simulink model "IEEE30_case"  (R2024b)
settings: Solver=FixedStepAuto  StartTime=0  StopTime=5  FixedStep=1e-7  RelTol=1e-3
values from neighbouring files (symbols this model uses):
  GFL_DFIG_7_C_bus = 0.08    [IEEE30_case_parameters.m]
  GFL_DFIG_7_D_mutual = 2.500000e+3    (= 2500)    [IEEE30_case_parameters.m]
  GFL_DFIG_7_f0 = 60    [IEEE30_case_parameters.m]
  GFL_DFIG_7_gPLLi = 3200    [IEEE30_case_parameters.m]
  GFL_DFIG_7_gPLLp = 650    [IEEE30_case_parameters.m]
  GFL_DFIG_7_H_WT = 0.4    [IEEE30_case_parameters.m]
  GFL_DFIG_7_Hg = 0.8    [IEEE30_case_parameters.m]
  GFL_DFIG_7_Igq_ref = 0    [IEEE30_case_parameters.m]
  GFL_DFIG_7_Ird_ref = 704.45696    [IEEE30_case_parameters.m]
  GFL_DFIG_7_KI_V = -300000    [IEEE30_case_parameters.m]
  GFL_DFIG_7_KP_V = -1000    [IEEE30_case_parameters.m]
  GFL_DFIG_7_Ksh = 1.254300e+4    (= 12543)    [IEEE30_case_parameters.m]
  GFL_DFIG_7_Lg = 0.000483    [IEEE30_case_parameters.m]
  GFL_DFIG_7_Lm_pu = 4    [IEEE30_case_parameters.m]
  GFL_DFIG_7_N = 100    [IEEE30_case_parameters.m]
  GFL_DFIG_7_p = 2    [IEEE30_case_parameters.m]
  GFL_DFIG_7_Pitch = 0    [IEEE30_case_parameters.m]
  GFL_DFIG_7_R = 44    [IEEE30_case_parameters.m]
  GFL_DFIG_7_Rg = 2.000000e-5    (= 2e-05)    [IEEE30_case_parameters.m]
  GFL_DFIG_7_rho = 1.225    [IEEE30_case_parameters.m]
  GFL_DFIG_7_rPLLi = 4500    [IEEE30_case_parameters.m]
  GFL_DFIG_7_rPLLp = 620    [IEEE30_case_parameters.m]
  GFL_DFIG_7_Rs_pu = 0.011    [IEEE30_case_parameters.m]
  GFL_DFIG_7_Sbase = 2.000000e+6    (= 2000000)    [IEEE30_case_parameters.m]
  GFL_DFIG_7_ugq_ref = 0    [IEEE30_case_parameters.m]
  GFL_DFIG_7_usd_ref = 0    [IEEE30_case_parameters.m]
  GFL_DFIG_7_Vbase = 690    [IEEE30_case_parameters.m]
  GFL_DFIG_7_Vdc_ref = 1200    [IEEE30_case_parameters.m]
  GFL_DFIG_7_wind = 12    [IEEE30_case_parameters.m]
  GFL_DFIG_7_wm_ref = 518.184209    [IEEE30_case_parameters.m]
  SG_D_13_D = 0.01056    [IEEE30_case_parameters.m]
  SG_D_13_EnableSaturation = 0    [IEEE30_case_parameters.m]
  SG_D_13_f0 = 60    [IEEE30_case_parameters.m]
  SG_D_13_H = 7.5    [IEEE30_case_parameters.m]
  SG_D_13_K_A = 20    [IEEE30_case_parameters.m]
  SG_D_13_K_E = 1.000000e+1    (= 10)    [IEEE30_case_parameters.m]
  SG_D_13_K_F = 2.363    [IEEE30_case_parameters.m]
  SG_D_13_K_s = 0.5    [IEEE30_case_parameters.m]
  SG_D_13_R_a = 0.001088    [IEEE30_case_parameters.m]
  SG_D_13_S_A = 1    [IEEE30_case_parameters.m]
  SG_D_13_S_B = 0.103    [IEEE30_case_parameters.m]
  SG_D_13_S_N = 10.659857    [IEEE30_case_parameters.m]
  SG_D_13_SpeedPara = 200    [IEEE30_case_parameters.m]
  SG_D_13_T_0 = 0.370163    [IEEE30_case_parameters.m]
  SG_D_13_T_1 = 0.3    [IEEE30_case_parameters.m]
  SG_D_13_T_2 = 0.05    [IEEE30_case_parameters.m]
  SG_D_13_T_3 = 0.02    [IEEE30_case_parameters.m]
  SG_D_13_T_4 = 0.005    [IEEE30_case_parameters.m]
  SG_D_13_T_A = 0.02    [IEEE30_case_parameters.m]
  SG_D_13_T_dd = 8.000000e+0    (= 8)    [IEEE30_case_parameters.m]
  SG_D_13_T_ddd = 0.04    [IEEE30_case_parameters.m]
  SG_D_13_T_E = 0.314    [IEEE30_case_parameters.m]
  SG_D_13_T_F = 0.35    [IEEE30_case_parameters.m]
  SG_D_13_T_qd = 0.8    [IEEE30_case_parameters.m]
  SG_D_13_T_qdd = 0.02    [IEEE30_case_parameters.m]
  SG_D_13_T_speed = 0.1    [IEEE30_case_parameters.m]
  SG_D_13_T_w = 0.5    [IEEE30_case_parameters.m]
  SG_D_13_V_ref = 1.696619    [IEEE30_case_parameters.m]
  SG_D_13_w_ref = 376.991118    [IEEE30_case_parameters.m]
  SG_D_13_x_d = 1.9    [IEEE30_case_parameters.m]
  SG_D_13_x_dd = 0.302    [IEEE30_case_parameters.m]
  SG_D_13_x_ddd = 0.204    [IEEE30_case_parameters.m]
  SG_D_13_x_l = 0.05    [IEEE30_case_parameters.m]
  SG_D_13_x_q = 1.3    [IEEE30_case_parameters.m]
  SG_D_13_x_qd = 0.5    [IEEE30_case_parameters.m]
  SG_D_13_x_qdd = 0.3    [IEEE30_case_parameters.m]
  SG_D_1_D = 0.01056    [IEEE30_case_parameters.m]
  SG_D_1_EnableSaturation = 0    [IEEE30_case_parameters.m]
  SG_D_1_f0 = 60    [IEEE30_case_parameters.m]
  SG_D_1_H = 7.5    [IEEE30_case_parameters.m]
  SG_D_1_K_A = 20    [IEEE30_case_parameters.m]
  SG_D_1_K_E = 1.000000e+1    (= 10)    [IEEE30_case_parameters.m]
  SG_D_1_K_F = 2.363    [IEEE30_case_parameters.m]
  SG_D_1_K_s = 0.5    [IEEE30_case_parameters.m]
  SG_D_1_R_a = 0.001088    [IEEE30_case_parameters.m]
  SG_D_1_S_A = 1    [IEEE30_case_parameters.m]
  SG_D_1_S_B = 0.103    [IEEE30_case_parameters.m]
  SG_D_1_S_N = 10.659857    [IEEE30_case_parameters.m]
  SG_D_1_SpeedPara = 200    [IEEE30_case_parameters.m]
  SG_D_1_T_0 = 0.259812    [IEEE30_case_parameters.m]
  SG_D_1_T_1 = 0.3    [IEEE30_case_parameters.m]
  SG_D_1_T_2 = 0.05    [IEEE30_case_parameters.m]
  SG_D_1_T_3 = 0.02    [IEEE30_case_parameters.m]
  SG_D_1_T_4 = 0.005    [IEEE30_case_parameters.m]
  SG_D_1_T_A = 0.02    [IEEE30_case_parameters.m]
  SG_D_1_T_dd = 8.000000e+0    (= 8)    [IEEE30_case_parameters.m]
  SG_D_1_T_ddd = 0.04    [IEEE30_case_parameters.m]
  SG_D_1_T_E = 0.314    [IEEE30_case_parameters.m]
  SG_D_1_T_F = 0.35    [IEEE30_case_parameters.m]
  SG_D_1_T_qd = 0.8    [IEEE30_case_parameters.m]
  SG_D_1_T_qdd = 0.02    [IEEE30_case_parameters.m]
  SG_D_1_T_speed = 0.1    [IEEE30_case_parameters.m]
  SG_D_1_T_w = 0.5    [IEEE30_case_parameters.m]
  SG_D_1_V_ref = 1.544107    [IEEE30_case_parameters.m]
  SG_D_1_w_ref = 376.991118    [IEEE30_case_parameters.m]
  SG_D_1_x_d = 1.9    [IEEE30_case_parameters.m]
  SG_D_1_x_dd = 0.302    [IEEE30_case_parameters.m]
  SG_D_1_x_ddd = 0.204    [IEEE30_case_parameters.m]
  SG_D_1_x_l = 0.05    [IEEE30_case_parameters.m]
  SG_D_1_x_q = 1.3    [IEEE30_case_parameters.m]
  SG_D_1_x_qd = 0.5    [IEEE30_case_parameters.m]
  SG_D_1_x_qdd = 0.3    [IEEE30_case_parameters.m]
  SG_D_22_D = 0.01056    [IEEE30_case_parameters.m]
  SG_D_22_EnableSaturation = 0    [IEEE30_case_parameters.m]
  SG_D_22_f0 = 60    [IEEE30_case_parameters.m]
  SG_D_22_H = 7.5    [IEEE30_case_parameters.m]
  SG_D_22_K_A = 20    [IEEE30_case_parameters.m]
  SG_D_22_K_E = 1.000000e+1    (= 10)    [IEEE30_case_parameters.m]
  SG_D_22_K_F = 2.363    [IEEE30_case_parameters.m]
  SG_D_22_K_s = 0.5    [IEEE30_case_parameters.m]
  SG_D_22_R_a = 0.001088    [IEEE30_case_parameters.m]
  SG_D_22_S_A = 1    [IEEE30_case_parameters.m]
  SG_D_22_S_B = 0.103    [IEEE30_case_parameters.m]
  SG_D_22_S_N = 10.659857    [IEEE30_case_parameters.m]
  SG_D_22_SpeedPara = 200    [IEEE30_case_parameters.m]
  SG_D_22_T_0 = 0.216121    [IEEE30_case_parameters.m]
  SG_D_22_T_1 = 0.3    [IEEE30_case_parameters.m]
  SG_D_22_T_2 = 0.05    [IEEE30_case_parameters.m]
  SG_D_22_T_3 = 0.02    [IEEE30_case_parameters.m]
  SG_D_22_T_4 = 0.005    [IEEE30_case_parameters.m]
  ... (+126 more)
(part 8 of 27)

== system IEEE30_case/AC_1/d_iq_line_2_5_block ==
  note: d_iq_line_2_5 in IEEE30_case
      | $1884.95559215388\,\mathrm{vq}_{\mathrm{bus},2}-94.2477796076938\,\mathrm{iq}_{\mathrm{line},2,5}-376.991118430775\,\mathrm{id}_{\mathrm{line},2,5}-1884.95559215388\,\mathrm{vq}_{\mathrm{bus},5}$
      | Automatically generated on 2025-11-01 18:41:07 .
  State_id_line_2_5_54524 : Inport
  State_iq_line_2_5_e8b89 : Inport  Port=2
  State_vq_bus_2_03b90 : Inport  Port=3
  State_vq_bus_5_87317 : Inport  Port=4
  Add_a371a : Sum
  Constant_-376.991118430775_afe3f : Constant  Value=-376.991118430775
  Constant_1884.95559215388_7223d : Constant  Value=1884.95559215388
  Constant_1884.95559215388_7e2ac : Constant  Value=1884.95559215388
  Constant_94.2477796076938_c5ea2 : Constant  Value=94.2477796076938
  Product_7cc1a : Product
  Product_8b282 : Product
  Product_c2d6a : Product
  Product_f29d2 : Product
  Subtract_19345 : Sum  Inputs=+-
  Subtract_26d55 : Sum  Inputs=+-
  Blockout_d_iq_line_2_5_eff7c : Outport
  wires:
  Constant_-376.991118430775_afe3f/1 -> Product_7cc1a/1
  Product_7cc1a/1 -> Subtract_26d55/1
  State_id_line_2_5_54524/1 -> Product_7cc1a/2
  Constant_94.2477796076938_c5ea2/1 -> Product_f29d2/1
  State_iq_line_2_5_e8b89/1 -> Product_f29d2/2
  Product_f29d2/1 -> Subtract_26d55/2
  State_vq_bus_2_03b90/1 -> Product_c2d6a/2
  Product_c2d6a/1 -> Add_a371a/2
  Constant_1884.95559215388_7223d/1 -> Product_c2d6a/1
  Subtract_26d55/1 -> Add_a371a/1
  Product_8b282/1 -> Subtract_19345/2
  Constant_1884.95559215388_7e2ac/1 -> Product_8b282/1
  State_vq_bus_5_87317/1 -> Product_8b282/2
  Add_a371a/1 -> Subtract_19345/1
  Subtract_19345/1 -> Blockout_d_iq_line_2_5_eff7c/1

== system IEEE30_case/AC_1/d_iq_line_2_6_block ==
  note: d_iq_line_2_6 in IEEE30_case
      | $2094.39510239319\,\mathrm{vq}_{\mathrm{bus},2}-125.663706143592\,\mathrm{iq}_{\mathrm{line},2,6}-376.991118430775\,\mathrm{id}_{\mathrm{line},2,6}-2094.39510239319\,\mathrm{vq}_{\mathrm{bus},6}$
      | Automatically generated on 2025-11-01 18:41:10 .
  State_id_line_2_6_7b42f : Inport
  State_iq_line_2_6_17b05 : Inport  Port=2
  State_vq_bus_2_0704f : Inport  Port=3
  State_vq_bus_6_e98dc : Inport  Port=4
  Add_94bf2 : Sum
  Constant_-376.991118430775_61c83 : Constant  Value=-376.991118430775
  Constant_125.663706143592_83d9a : Constant  Value=125.663706143592
  Constant_2094.39510239319_5703c : Constant  Value=2094.39510239319
  Constant_2094.39510239319_adbae : Constant  Value=2094.39510239319
  Product_1e63b : Product
  Product_508a7 : Product
  Product_89e1e : Product
  Product_db02a : Product
  Subtract_5e54d : Sum  Inputs=+-
  Subtract_f5901 : Sum  Inputs=+-
  Blockout_d_iq_line_2_6_890b3 : Outport
  wires:
  Constant_-376.991118430775_61c83/1 -> Product_508a7/1
  State_id_line_2_6_7b42f/1 -> Product_508a7/2
  Constant_125.663706143592_83d9a/1 -> Product_db02a/1
  Product_db02a/1 -> Subtract_f5901/2
  Product_89e1e/1 -> Add_94bf2/2
  Constant_2094.39510239319_5703c/1 -> Product_89e1e/1
  State_iq_line_2_6_17b05/1 -> Product_db02a/2
  Product_508a7/1 -> Subtract_f5901/1
  State_vq_bus_2_0704f/1 -> Product_89e1e/2
  Subtract_f5901/1 -> Add_94bf2/1
  Product_1e63b/1 -> Subtract_5e54d/2
  Constant_2094.39510239319_adbae/1 -> Product_1e63b/1
  Add_94bf2/1 -> Subtract_5e54d/1
  State_vq_bus_6_e98dc/1 -> Product_1e63b/2
  Subtract_5e54d/1 -> Blockout_d_iq_line_2_6_890b3/1

== system IEEE30_case/AC_1/d_iq_line_3_4_block ==
  note: d_iq_line_3_4 in IEEE30_case
      | $9424.77796076938\,\mathrm{vq}_{\mathrm{bus},3}-94.2477796076938\,\mathrm{iq}_{\mathrm{line},3,4}-376.991118430775\,\mathrm{id}_{\mathrm{line},3,4}-9424.77796076938\,\mathrm{vq}_{\mathrm{bus},4}$
      | Automatically generated on 2025-11-01 18:41:05 .
  State_id_line_3_4_c2377 : Inport
  State_iq_line_3_4_a2132 : Inport  Port=2
  State_vq_bus_3_53dc7 : Inport  Port=3
  State_vq_bus_4_f5988 : Inport  Port=4
  Add_93964 : Sum
  Constant_-376.991118430775_c7e30 : Constant  Value=-376.991118430775
  Constant_94.2477796076938_a3062 : Constant  Value=94.2477796076938
  Constant_9424.77796076938_25937 : Constant  Value=9424.77796076938
  Constant_9424.77796076938_71653 : Constant  Value=9424.77796076938
  Product_1bd2b : Product
  Product_9bcd3 : Product
  Product_bb908 : Product
  Product_e88d9 : Product
  Subtract_42a0d : Sum  Inputs=+-
  Subtract_80c72 : Sum  Inputs=+-
  Blockout_d_iq_line_3_4_9b5ec : Outport
  wires:
  Constant_-376.991118430775_c7e30/1 -> Product_9bcd3/1
  Constant_94.2477796076938_a3062/1 -> Product_1bd2b/1
  Product_1bd2b/1 -> Subtract_42a0d/2
  Product_9bcd3/1 -> Subtract_42a0d/1
  State_id_line_3_4_c2377/1 -> Product_9bcd3/2
  State_iq_line_3_4_a2132/1 -> Product_1bd2b/2
  Product_bb908/1 -> Add_93964/2
  Constant_9424.77796076938_71653/1 -> Product_bb908/1
  State_vq_bus_3_53dc7/1 -> Product_bb908/2
  Product_e88d9/1 -> Subtract_80c72/2
  Subtract_42a0d/1 -> Add_93964/1
  Constant_9424.77796076938_25937/1 -> Product_e88d9/1
  State_vq_bus_4_f5988/1 -> Product_e88d9/2
  Add_93964/1 -> Subtract_80c72/1
  Subtract_80c72/1 -> Blockout_d_iq_line_3_4_9b5ec/1

== system IEEE30_case/AC_1/d_iq_line_4_12_block ==
  note: d_iq_line_4_12 in IEEE30_case
      | $1449.96584011837\,\mathrm{vq}_{\mathrm{bus},4}-376.991118430775\,\mathrm{id}_{\mathrm{line},4,12}-1449.96584011837\,\mathrm{vq}_{\mathrm{bus},12}$
      | Automatically generated on 2025-11-01 18:41:30 .
  State_id_line_4_12_e9a32 : Inport
  State_vq_bus_12_318e0 : Inport  Port=2
  State_vq_bus_4_bbada : Inport  Port=3
  Add_42926 : Sum
  Constant_-376.991118430775_8ab2d : Constant  Value=-376.991118430775
  Constant_1449.96584011837_54b12 : Constant  Value=1449.96584011837
  Constant_1449.96584011837_d2e29 : Constant  Value=1449.96584011837
  Product_7ffdd : Product
  Product_e5260 : Product
  Product_e61c8 : Product
  Subtract_d7829 : Sum  Inputs=+-
  Blockout_d_iq_line_4_12_9b276 : Outport
  wires:
  Constant_-376.991118430775_8ab2d/1 -> Product_7ffdd/1
  Constant_1449.96584011837_54b12/1 -> Product_e5260/1
  Product_e5260/1 -> Subtract_d7829/2
  Product_7ffdd/1 -> Subtract_d7829/1
  State_id_line_4_12_e9a32/1 -> Product_7ffdd/2
  State_vq_bus_12_318e0/1 -> Product_e5260/2
  Product_e61c8/1 -> Add_42926/2
  Constant_1449.96584011837_d2e29/1 -> Product_e61c8/1
  Add_42926/1 -> Blockout_d_iq_line_4_12_9b276/1
  State_vq_bus_4_bbada/1 -> Product_e61c8/2
  Subtract_d7829/1 -> Add_42926/1

== system IEEE30_case/AC_1/d_iq_line_4_6_block ==
  note: d_iq_line_4_6 in IEEE30_case
      | $9424.77796076938\,\mathrm{vq}_{\mathrm{bus},4}-94.2477796076938\,\mathrm{iq}_{\mathrm{line},4,6}-376.991118430775\,\mathrm{id}_{\mathrm{line},4,6}-9424.77796076938\,\mathrm{vq}_{\mathrm{bus},6}$
      | Automatically generated on 2025-11-01 18:41:12 .
  State_id_line_4_6_aad9c : Inport
  State_iq_line_4_6_338ba : Inport  Port=2
  State_vq_bus_4_bd5e4 : Inport  Port=3
  State_vq_bus_6_b2fe0 : Inport  Port=4
  Add_f3899 : Sum
  Constant_-376.991118430775_1ade0 : Constant  Value=-376.991118430775
  Constant_94.2477796076938_b364f : Constant  Value=94.2477796076938
  Constant_9424.77796076938_20b18 : Constant  Value=9424.77796076938
  Constant_9424.77796076938_69e60 : Constant  Value=9424.77796076938
  Product_28995 : Product
  Product_5675d : Product
  Product_6de9b : Product
  Product_811d8 : Product
  Subtract_07f3b : Sum  Inputs=+-
  Subtract_17cad : Sum  Inputs=+-
  Blockout_d_iq_line_4_6_3cc9a : Outport
  wires:
  State_iq_line_4_6_338ba/1 -> Product_6de9b/2
  Constant_-376.991118430775_1ade0/1 -> Product_5675d/1
  Constant_94.2477796076938_b364f/1 -> Product_6de9b/1
  Product_6de9b/1 -> Subtract_07f3b/2
  State_id_line_4_6_aad9c/1 -> Product_5675d/2
  Product_5675d/1 -> Subtract_07f3b/1
  Constant_9424.77796076938_69e60/1 -> Product_28995/1
  State_vq_bus_4_bd5e4/1 -> Product_28995/2
  Subtract_07f3b/1 -> Add_f3899/1
  Product_28995/1 -> Add_f3899/2
  Product_811d8/1 -> Subtract_17cad/2
  Constant_9424.77796076938_20b18/1 -> Product_811d8/1
  State_vq_bus_6_b2fe0/1 -> Product_811d8/2
  Add_f3899/1 -> Subtract_17cad/1
  Subtract_17cad/1 -> Blockout_d_iq_line_4_6_3cc9a/1

== system IEEE30_case/AC_1/d_iq_line_5_7_block ==
  note: d_iq_line_5_7 in IEEE30_case
      | $3141.59265358979\,\mathrm{vq}_{\mathrm{bus},5}-157.07963267949\,\mathrm{iq}_{\mathrm{line},5,7}-376.991118430775\,\mathrm{id}_{\mathrm{line},5,7}-3141.59265358979\,\mathrm{vq}_{\mathrm{bus},7}$
      | Automatically generated on 2025-11-01 18:41:15 .
  State_id_line_5_7_c3a9a : Inport
  State_iq_line_5_7_98783 : Inport  Port=2
  State_vq_bus_5_129b8 : Inport  Port=3
  State_vq_bus_7_b0dc6 : Inport  Port=4
  Add_6172d : Sum
  Constant_-376.991118430775_516df : Constant  Value=-376.991118430775
  Constant_157.07963267949_263dc : Constant  Value=157.07963267949
  Constant_3141.59265358979_47382 : Constant  Value=3141.59265358979
  Constant_3141.59265358979_720d9 : Constant  Value=3141.59265358979
  Product_25a26 : Product
  Product_4ad97 : Product
  Product_59bd4 : Product
  Product_d4615 : Product
  Subtract_670ee : Sum  Inputs=+-
  Subtract_989a0 : Sum  Inputs=+-
  Blockout_d_iq_line_5_7_5e840 : Outport
  wires:
  Constant_-376.991118430775_516df/1 -> Product_4ad97/1
  Product_4ad97/1 -> Subtract_670ee/1
  State_id_line_5_7_c3a9a/1 -> Product_4ad97/2
  Constant_157.07963267949_263dc/1 -> Product_59bd4/1
  Product_59bd4/1 -> Subtract_670ee/2
  State_iq_line_5_7_98783/1 -> Product_59bd4/2
  Product_25a26/1 -> Add_6172d/2
  Constant_3141.59265358979_720d9/1 -> Product_25a26/1
  State_vq_bus_5_129b8/1 -> Product_25a26/2
  Subtract_670ee/1 -> Add_6172d/1
  Constant_3141.59265358979_47382/1 -> Product_d4615/1
  State_vq_bus_7_b0dc6/1 -> Product_d4615/2
  Add_6172d/1 -> Subtract_989a0/1
  Product_d4615/1 -> Subtract_989a0/2
  Subtract_989a0/1 -> Blockout_d_iq_line_5_7_5e840/1

== system IEEE30_case/AC_1/d_iq_line_6_10_block ==
  note: d_iq_line_6_10 in IEEE30_case
      | $673.198425769241\,\mathrm{vq}_{\mathrm{bus},6}-376.991118430775\,\mathrm{id}_{\mathrm{line},6,10}-673.198425769241\,\mathrm{vq}_{\mathrm{bus},10}$
      | Automatically generated on 2025-11-01 18:41:24 .
  State_id_line_6_10_fd3de : Inport
  State_vq_bus_10_9c824 : Inport  Port=2
  State_vq_bus_6_fa482 : Inport  Port=3
  Add_8fad6 : Sum
  Constant_-376.991118430775_b3dc4 : Constant  Value=-376.991118430775
  Constant_673.198425769241_7fad7 : Constant  Value=673.198425769241
  Constant_673.198425769241_d3814 : Constant  Value=673.198425769241
  Product_129d7 : Product
  Product_6bf2e : Product
  Product_9f14d : Product
  Subtract_2b990 : Sum  Inputs=+-
  Blockout_d_iq_line_6_10_02488 : Outport
  wires:
  Constant_-376.991118430775_b3dc4/1 -> Product_129d7/1
  Product_129d7/1 -> Subtract_2b990/1
  State_id_line_6_10_fd3de/1 -> Product_129d7/2
  Constant_673.198425769241_d3814/1 -> Product_9f14d/1
  Product_9f14d/1 -> Subtract_2b990/2
  State_vq_bus_10_9c824/1 -> Product_9f14d/2
  Product_6bf2e/1 -> Add_8fad6/2
  Constant_673.198425769241_7fad7/1 -> Product_6bf2e/1
  State_vq_bus_6_fa482/1 -> Product_6bf2e/2
  Subtract_2b990/1 -> Add_8fad6/1
  Add_8fad6/1 -> Blockout_d_iq_line_6_10_02488/1

== system IEEE30_case/AC_1/d_iq_line_6_28_block ==
  note: d_iq_line_6_28 in IEEE30_case
      | $6283.18530717959\,\mathrm{vq}_{\mathrm{bus},6}-125.663706143592\,\mathrm{iq}_{\mathrm{line},6,28}-376.991118430775\,\mathrm{id}_{\mathrm{line},6,28}-6283.18530717959\,\mathrm{vq}_{\mathrm{bus},28}$
      | Automatically generated on 2025-11-01 18:42:31 .
  State_id_line_6_28_8e443 : Inport
  State_iq_line_6_28_bd7e8 : Inport  Port=2
  State_vq_bus_28_c063c : Inport  Port=3
  State_vq_bus_6_177ff : Inport  Port=4
  Add_6d067 : Sum
  Constant_-376.991118430775_906bc : Constant  Value=-376.991118430775
  Constant_125.663706143592_e6af5 : Constant  Value=125.663706143592
  Constant_6283.18530717959_22793 : Constant  Value=6283.18530717959
  Constant_6283.18530717959_eb312 : Constant  Value=6283.18530717959
  Product_0abd7 : Product
  Product_128c9 : Product
  Product_5e22f : Product
  Product_646a6 : Product
  Subtract_5dc35 : Sum  Inputs=+-
  Subtract_e4d26 : Sum  Inputs=+-
  Blockout_d_iq_line_6_28_5907d : Outport
  wires:
  State_id_line_6_28_8e443/1 -> Product_128c9/2
  Constant_-376.991118430775_906bc/1 -> Product_128c9/1
  Constant_125.663706143592_e6af5/1 -> Product_646a6/1
  Product_646a6/1 -> Subtract_5dc35/2
  State_iq_line_6_28_bd7e8/1 -> Product_646a6/2
  Product_128c9/1 -> Subtract_5dc35/1
  Product_0abd7/1 -> Subtract_e4d26/2
  Constant_6283.18530717959_22793/1 -> Product_0abd7/1
  State_vq_bus_28_c063c/1 -> Product_0abd7/2
  Subtract_5dc35/1 -> Subtract_e4d26/1
  Product_5e22f/1 -> Add_6d067/2
  Constant_6283.18530717959_eb312/1 -> Product_5e22f/1
  State_vq_bus_6_177ff/1 -> Product_5e22f/2
  Subtract_e4d26/1 -> Add_6d067/1
  Add_6d067/1 -> Blockout_d_iq_line_6_28_5907d/1

== system IEEE30_case/AC_1/d_iq_line_6_7_block ==
  note: d_iq_line_6_7 in IEEE30_case
      | $4712.38898038469\,\mathrm{vq}_{\mathrm{bus},6}-141.371669411541\,\mathrm{iq}_{\mathrm{line},6,7}-376.991118430775\,\mathrm{id}_{\mathrm{line},6,7}-4712.38898038469\,\mathrm{vq}_{\mathrm{bus},7}$
      | Automatically generated on 2025-11-01 18:41:17 .
  State_id_line_6_7_667e6 : Inport
  State_iq_line_6_7_562f8 : Inport  Port=2
  State_vq_bus_6_83d07 : Inport  Port=3
  State_vq_bus_7_9b0dd : Inport  Port=4
  Add_794fe : Sum
  Constant_-376.991118430775_81a88 : Constant  Value=-376.991118430775
  Constant_141.371669411541_92a0d : Constant  Value=141.371669411541
  Constant_4712.38898038469_6f32c : Constant  Value=4712.38898038469
  Constant_4712.38898038469_e9fde : Constant  Value=4712.38898038469
  Product_190ff : Product
  Product_32f70 : Product
  Product_ab4c4 : Product
  Product_ee51e : Product
  Subtract_10fa6 : Sum  Inputs=+-
  Subtract_c84df : Sum  Inputs=+-
  Blockout_d_iq_line_6_7_6dbe9 : Outport
  wires:
  Constant_-376.991118430775_81a88/1 -> Product_32f70/1
  Product_32f70/1 -> Subtract_10fa6/1
  State_id_line_6_7_667e6/1 -> Product_32f70/2
  Constant_141.371669411541_92a0d/1 -> Product_ee51e/1
  Product_190ff/1 -> Add_794fe/2
  Constant_4712.38898038469_6f32c/1 -> Product_190ff/1
  State_iq_line_6_7_562f8/1 -> Product_ee51e/2
  State_vq_bus_6_83d07/1 -> Product_190ff/2
  Product_ee51e/1 -> Subtract_10fa6/2
  Subtract_10fa6/1 -> Add_794fe/1
  Product_ab4c4/1 -> Subtract_c84df/2
  Constant_4712.38898038469_e9fde/1 -> Product_ab4c4/1
  State_vq_bus_7_9b0dd/1 -> Product_ab4c4/2
  Add_794fe/1 -> Subtract_c84df/1
  Subtract_c84df/1 -> Blockout_d_iq_line_6_7_6dbe9/1

== system IEEE30_case/AC_1/d_iq_line_6_8_block ==
  note: d_iq_line_6_8 in IEEE30_case
      | $9424.77796076938\,\mathrm{vq}_{\mathrm{bus},6}-94.2477796076938\,\mathrm{iq}_{\mathrm{line},6,8}-376.991118430775\,\mathrm{id}_{\mathrm{line},6,8}-9424.77796076938\,\mathrm{vq}_{\mathrm{bus},8}$
      | Automatically generated on 2025-11-01 18:41:19 .
  State_id_line_6_8_d622b : Inport
  State_iq_line_6_8_6bc9f : Inport  Port=2
  State_vq_bus_6_241ca : Inport  Port=3
  State_vq_bus_8_0df72 : Inport  Port=4
  Add_b3718 : Sum
  Constant_-376.991118430775_fad48 : Constant  Value=-376.991118430775
  Constant_94.2477796076938_eb35d : Constant  Value=94.2477796076938
  Constant_9424.77796076938_61207 : Constant  Value=9424.77796076938
  Constant_9424.77796076938_d91cc : Constant  Value=9424.77796076938
  Product_9a554 : Product
  Product_cf133 : Product
  Product_e540a : Product
  Product_ed09e : Product
  Subtract_a6489 : Sum  Inputs=+-
  Subtract_b0ec5 : Sum  Inputs=+-
  Blockout_d_iq_line_6_8_b8ba9 : Outport
  wires:
  Constant_-376.991118430775_fad48/1 -> Product_cf133/1
  Constant_94.2477796076938_eb35d/1 -> Product_e540a/1
  Product_e540a/1 -> Subtract_b0ec5/2
  State_id_line_6_8_d622b/1 -> Product_cf133/2
  State_iq_line_6_8_6bc9f/1 -> Product_e540a/2
  Product_9a554/1 -> Add_b3718/2
  Constant_9424.77796076938_61207/1 -> Product_9a554/1
  Product_cf133/1 -> Subtract_b0ec5/1
  State_vq_bus_6_241ca/1 -> Product_9a554/2
  Subtract_b0ec5/1 -> Add_b3718/1
  Product_ed09e/1 -> Subtract_a6489/2
  Constant_9424.77796076938_d91cc/1 -> Product_ed09e/1
  State_vq_bus_8_0df72/1 -> Product_ed09e/2
  Add_b3718/1 -> Subtract_a6489/1
  Subtract_a6489/1 -> Blockout_d_iq_line_6_8_b8ba9/1

== system IEEE30_case/AC_1/d_iq_line_6_9_block ==
  note: d_iq_line_6_9 in IEEE30_case
      | $1795.19580205131\,\mathrm{vq}_{\mathrm{bus},6}-376.991118430775\,\mathrm{id}_{\mathrm{line},6,9}-1795.19580205131\,\mathrm{vq}_{\mathrm{bus},9}$
      | Automatically generated on 2025-11-01 18:41:22 .
  State_id_line_6_9_7cf57 : Inport
  State_vq_bus_6_65d52 : Inport  Port=2
  State_vq_bus_9_a086b : Inport  Port=3
  Add_f6946 : Sum
  Constant_-376.991118430775_59e94 : Constant  Value=-376.991118430775
  Constant_1795.19580205131_6c4f5 : Constant  Value=1795.19580205131
  Constant_1795.19580205131_bd9ec : Constant  Value=1795.19580205131
  Product_09b80 : Product
  Product_17dc1 : Product
  Product_908ab : Product
  Subtract_cd50a : Sum  Inputs=+-
  Blockout_d_iq_line_6_9_e28b1 : Outport
  wires:
  Constant_-376.991118430775_59e94/1 -> Product_17dc1/1
  Constant_1795.19580205131_6c4f5/1 -> Product_908ab/1
  Product_908ab/1 -> Add_f6946/2
  Product_17dc1/1 -> Add_f6946/1
  State_id_line_6_9_7cf57/1 -> Product_17dc1/2
  State_vq_bus_6_65d52/1 -> Product_908ab/2
  Product_09b80/1 -> Subtract_cd50a/2
  Constant_1795.19580205131_bd9ec/1 -> Product_09b80/1
  Subtract_cd50a/1 -> Blockout_d_iq_line_6_9_e28b1/1
  State_vq_bus_9_a086b/1 -> Product_09b80/2
  Add_f6946/1 -> Subtract_cd50a/1

== system IEEE30_case/AC_1/d_iq_line_8_28_block ==
  note: d_iq_line_8_28 in IEEE30_case
      | $1884.95559215388\,\mathrm{vq}_{\mathrm{bus},8}-113.097335529233\,\mathrm{iq}_{\mathrm{line},8,28}-376.991118430775\,\mathrm{id}_{\mathrm{line},8,28}-1884.95559215388\,\mathrm{vq}_{\mathrm{bus},28}$
      | Automatically generated on 2025-11-01 18:42:28 .
  State_id_line_8_28_812ec : Inport
  State_iq_line_8_28_65df2 : Inport  Port=2
  State_vq_bus_28_2fdab : Inport  Port=3
  State_vq_bus_8_f157d : Inport  Port=4
  Add_148f8 : Sum
  Constant_-376.991118430775_e146a : Constant  Value=-376.991118430775
  Constant_113.097335529233_20841 : Constant  Value=113.097335529233
  Constant_1884.95559215388_0a6d6 : Constant  Value=1884.95559215388
  Constant_1884.95559215388_3768c : Constant  Value=1884.95559215388
  Product_312c0 : Product
  Product_51235 : Product
  Product_960d5 : Product
  Product_b56d3 : Product
  Subtract_9c826 : Sum  Inputs=+-
  Subtract_beca7 : Sum  Inputs=+-
  Blockout_d_iq_line_8_28_1c551 : Outport
  wires:
  Constant_-376.991118430775_e146a/1 -> Product_51235/1
  Product_960d5/1 -> Subtract_9c826/2
  Constant_1884.95559215388_0a6d6/1 -> Product_960d5/1
  Product_51235/1 -> Subtract_beca7/1
  State_id_line_8_28_812ec/1 -> Product_51235/2
  Constant_113.097335529233_20841/1 -> Product_312c0/1
  Product_312c0/1 -> Subtract_beca7/2
  State_iq_line_8_28_65df2/1 -> Product_312c0/2
  State_vq_bus_28_2fdab/1 -> Product_960d5/2
  Subtract_beca7/1 -> Subtract_9c826/1
  Product_b56d3/1 -> Add_148f8/2
  Constant_1884.95559215388_3768c/1 -> Product_b56d3/1
  State_vq_bus_8_f157d/1 -> Product_b56d3/2
  Subtract_9c826/1 -> Add_148f8/1
  Add_148f8/1 -> Blockout_d_iq_line_8_28_1c551/1

== system IEEE30_case/AC_1/d_iq_line_9_10_block ==
  note: d_iq_line_9_10 in IEEE30_case
      | $3427.19198573432\,\mathrm{vq}_{\mathrm{bus},9}-376.991118430775\,\mathrm{id}_{\mathrm{line},9,10}-3427.19198573432\,\mathrm{vq}_{\mathrm{bus},10}$
      | Automatically generated on 2025-11-01 18:41:28 .
  State_id_line_9_10_9405b : Inport
  State_vq_bus_10_72139 : Inport  Port=2
  State_vq_bus_9_3ff0d : Inport  Port=3
  Add_264a1 : Sum
  Constant_-376.991118430775_5d75f : Constant  Value=-376.991118430775
  Constant_3427.19198573432_1f815 : Constant  Value=3427.19198573432
  Constant_3427.19198573432_58760 : Constant  Value=3427.19198573432
  Product_adb61 : Product
  Product_c8172 : Product
  Product_ef6f6 : Product
  Subtract_5c677 : Sum  Inputs=+-
  Blockout_d_iq_line_9_10_d1a46 : Outport
  wires:
  State_vq_bus_9_3ff0d/1 -> Product_c8172/2
  Constant_-376.991118430775_5d75f/1 -> Product_ef6f6/1
  Product_c8172/1 -> Add_264a1/2
  Product_ef6f6/1 -> Subtract_5c677/1
  Constant_3427.19198573432_1f815/1 -> Product_c8172/1
  State_id_line_9_10_9405b/1 -> Product_ef6f6/2
  Constant_3427.19198573432_58760/1 -> Product_adb61/1
  State_vq_bus_10_72139/1 -> Product_adb61/2
  Product_adb61/1 -> Subtract_5c677/2
  Subtract_5c677/1 -> Add_264a1/1
  Add_264a1/1 -> Blockout_d_iq_line_9_10_d1a46/1

== system IEEE30_case/AC_1/d_iq_line_9_11_block ==
  note: d_iq_line_9_11 in IEEE30_case
      | $1795.19580205131\,\mathrm{vq}_{\mathrm{bus},9}-376.991118430775\,\mathrm{id}_{\mathrm{line},9,11}-1795.19580205131\,\mathrm{vq}_{\mathrm{bus},11}$
      | Automatically generated on 2025-11-01 18:41:26 .
  State_id_line_9_11_716ef : Inport
  State_vq_bus_11_310c2 : Inport  Port=2
  State_vq_bus_9_0d25d : Inport  Port=3
  Add_3daa9 : Sum
  Constant_-376.991118430775_ec185 : Constant  Value=-376.991118430775
  Constant_1795.19580205131_3f8cc : Constant  Value=1795.19580205131
  Constant_1795.19580205131_4c27b : Constant  Value=1795.19580205131
  Product_0918f : Product
  Product_28f02 : Product
  Product_341b4 : Product
  Subtract_55c47 : Sum  Inputs=+-
  Blockout_d_iq_line_9_11_ec45f : Outport
  wires:
  Constant_-376.991118430775_ec185/1 -> Product_0918f/1
  Product_0918f/1 -> Subtract_55c47/1
  State_id_line_9_11_716ef/1 -> Product_0918f/2
  Constant_1795.19580205131_3f8cc/1 -> Product_28f02/1
  Product_28f02/1 -> Subtract_55c47/2
  Product_341b4/1 -> Add_3daa9/2
  Constant_1795.19580205131_4c27b/1 -> Product_341b4/1
  State_vq_bus_11_310c2/1 -> Product_28f02/2
  State_vq_bus_9_0d25d/1 -> Product_341b4/2
  Subtract_55c47/1 -> Add_3daa9/1
  Add_3daa9/1 -> Blockout_d_iq_line_9_11_ec45f/1

== system IEEE30_case/AC_1/d_iq_load_10_block ==
  note: d_iq_load_10 in IEEE30_case
      | $73.2156181903037\,\mathrm{vq}_{\mathrm{bus},10}-1093.27424344925\,\mathrm{iq}_{\mathrm{load},10}-376.991118430775\,\mathrm{id}_{\mathrm{load},10}$
      | Automatically generated on 2025-11-01 18:40:26 .
  State_id_load_10_13915 : Inport
  State_iq_load_10_267fb : Inport  Port=2
  State_vq_bus_10_c6f4b : Inport  Port=3
  Add_9bcc7 : Sum
  Constant_-376.991118430775_f4f50 : Constant  Value=-376.991118430775
  Constant_1093.27424344925_5db7f : Constant  Value=1093.27424344925
  Constant_73.2156181903037_815ec : Constant  Value=73.2156181903037
  Product_7e589 : Product
  Product_b1673 : Product
  Product_faef5 : Product
  Subtract_39713 : Sum  Inputs=+-
  Blockout_d_iq_load_10_a5f74 : Outport
  wires:
  Constant_-376.991118430775_f4f50/1 -> Product_faef5/1
  Constant_73.2156181903037_815ec/1 -> Product_b1673/1
  State_id_load_10_13915/1 -> Product_faef5/2
  Constant_1093.27424344925_5db7f/1 -> Product_7e589/1
  Product_7e589/1 -> Subtract_39713/2
  State_iq_load_10_267fb/1 -> Product_7e589/2
  Product_faef5/1 -> Subtract_39713/1
  State_vq_bus_10_c6f4b/1 -> Product_b1673/2
  Subtract_39713/1 -> Add_9bcc7/1
  Product_b1673/1 -> Add_9bcc7/2
  Add_9bcc7/1 -> Blockout_d_iq_load_10_a5f74/1

== system IEEE30_case/AC_1/d_iq_load_12_block ==
  note: d_iq_load_12 in IEEE30_case
      | $94.0406333232708\,\mathrm{vq}_{\mathrm{bus},12}-562.973403523291\,\mathrm{iq}_{\mathrm{load},12}-376.991118430775\,\mathrm{id}_{\mathrm{load},12}$
      | Automatically generated on 2025-11-01 18:40:28 .
  State_id_load_12_a9fac : Inport
  State_iq_load_12_0eed2 : Inport  Port=2
  State_vq_bus_12_ac2a3 : Inport  Port=3
  Add_91925 : Sum
  Constant_-376.991118430775_6100e : Constant  Value=-376.991118430775
  Constant_562.973403523291_a5745 : Constant  Value=562.973403523291
  Constant_94.0406333232708_6cdec : Constant  Value=94.0406333232708
  Product_cf934 : Product
  Product_d0b54 : Product
  Product_e8b5c : Product
  Subtract_c298b : Sum  Inputs=+-
  Blockout_d_iq_load_12_fd87b : Outport
  wires:
  Constant_-376.991118430775_6100e/1 -> Product_e8b5c/1
  Constant_562.973403523291_a5745/1 -> Product_d0b54/1
  Product_d0b54/1 -> Subtract_c298b/2
  State_id_load_12_a9fac/1 -> Product_e8b5c/2
  State_iq_load_12_0eed2/1 -> Product_d0b54/2
  Product_e8b5c/1 -> Subtract_c298b/1
  Constant_94.0406333232708_6cdec/1 -> Product_cf934/1
  State_vq_bus_12_ac2a3/1 -> Product_cf934/2
  Subtract_c298b/1 -> Add_91925/1
  Product_cf934/1 -> Add_91925/2
  Add_91925/1 -> Blockout_d_iq_load_12_fd87b/1

== system IEEE30_case/AC_1/d_iq_load_14_block ==
  note: d_iq_load_14 in IEEE30_case
      | $101.272894526084\,\mathrm{vq}_{\mathrm{bus},14}-1460.84058391925\,\mathrm{iq}_{\mathrm{load},14}-376.991118430775\,\mathrm{id}_{\mathrm{load},14}$
      | Automatically generated on 2025-11-01 18:40:31 .
  State_id_load_14_258e7 : Inport
  State_iq_load_14_32f4c : Inport  Port=2
  State_vq_bus_14_0c5a3 : Inport  Port=3
  Add_63ca6 : Sum
  Constant_-376.991118430775_c30c3 : Constant  Value=-376.991118430775
  Constant_101.272894526084_db1b1 : Constant  Value=101.272894526084
  Constant_1460.84058391925_06af2 : Constant  Value=1460.84058391925
  Product_91f16 : Product
  Product_969e2 : Product
  Product_a0568 : Product
  Subtract_fed73 : Sum  Inputs=+-
  Blockout_d_iq_load_14_e1c59 : Outport
  wires:
  State_id_load_14_258e7/1 -> Product_969e2/2
  Constant_-376.991118430775_c30c3/1 -> Product_969e2/1
  Constant_1460.84058391925_06af2/1 -> Product_91f16/1
  Product_91f16/1 -> Subtract_fed73/2
  State_iq_load_14_32f4c/1 -> Product_91f16/2
  Product_969e2/1 -> Subtract_fed73/1
  Constant_101.272894526084_db1b1/1 -> Product_a0568/1
  State_vq_bus_14_0c5a3/1 -> Product_a0568/2
  Subtract_fed73/1 -> Add_63ca6/1
  Product_a0568/1 -> Add_63ca6/2
  Add_63ca6/1 -> Blockout_d_iq_load_14_e1c59/1

== system IEEE30_case/AC_1/d_iq_load_15_block ==
  note: d_iq_load_15 in IEEE30_case
      | $115.335827789783\,\mathrm{vq}_{\mathrm{bus},15}-1236.53086845294\,\mathrm{iq}_{\mathrm{load},15}-376.991118430775\,\mathrm{id}_{\mathrm{load},15}$
      | Automatically generated on 2025-11-01 18:40:33 .
  State_id_load_15_529a5 : Inport
  State_iq_load_15_0f08a : Inport  Port=2
  State_vq_bus_15_9de62 : Inport  Port=3
  Add_cd18a : Sum
  Constant_-376.991118430775_b8f9e : Constant  Value=-376.991118430775
  Constant_115.335827789783_f0de2 : Constant  Value=115.335827789783
  Constant_1236.53086845294_ddcf3 : Constant  Value=1236.53086845294
  Product_24c1c : Product
  Product_e4fc8 : Product
  Product_f8424 : Product
  Subtract_891f8 : Sum  Inputs=+-
  Blockout_d_iq_load_15_d1c82 : Outport
  wires:
  Constant_-376.991118430775_b8f9e/1 -> Product_f8424/1
  State_id_load_15_529a5/1 -> Product_f8424/2
  Constant_1236.53086845294_ddcf3/1 -> Product_24c1c/1
  Product_24c1c/1 -> Subtract_891f8/2
  State_iq_load_15_0f08a/1 -> Product_24c1c/2
  Product_f8424/1 -> Subtract_891f8/1
  Constant_115.335827789783_f0de2/1 -> Product_e4fc8/1
  State_vq_bus_15_9de62/1 -> Product_e4fc8/2
  Subtract_891f8/1 -> Add_cd18a/1
  Product_e4fc8/1 -> Add_cd18a/2
  Add_cd18a/1 -> Blockout_d_iq_load_15_d1c82/1

== system IEEE30_case/AC_1/d_iq_load_16_block ==
  note: d_iq_load_16 in IEEE30_case
      | $33.9601202098734\,\mathrm{vq}_{\mathrm{bus},16}-733.038285837618\,\mathrm{iq}_{\mathrm{load},16}-376.991118430775\,\mathrm{id}_{\mathrm{load},16}$
      | Automatically generated on 2025-11-01 18:40:35 .
  State_id_load_16_bee16 : Inport
  State_iq_load_16_5f7c5 : Inport  Port=2
  State_vq_bus_16_c51f8 : Inport  Port=3
  Add_8dc90 : Sum
  Constant_-376.991118430775_4be04 : Constant  Value=-376.991118430775
  Constant_33.9601202098734_a71af : Constant  Value=33.9601202098734
  Constant_733.038285837618_846d7 : Constant  Value=733.038285837618
  Product_11f64 : Product
  Product_a999c : Product
  Product_ec6fc : Product
  Subtract_5712a : Sum  Inputs=+-
  Blockout_d_iq_load_16_0762f : Outport
  wires:
  Constant_-376.991118430775_4be04/1 -> Product_a999c/1
  Constant_33.9601202098734_a71af/1 -> Product_ec6fc/1
  State_id_load_16_bee16/1 -> Product_a999c/2
  Constant_733.038285837618_846d7/1 -> Product_11f64/1
  Product_11f64/1 -> Subtract_5712a/2
  State_iq_load_16_5f7c5/1 -> Product_11f64/2
  Product_a999c/1 -> Subtract_5712a/1
  State_vq_bus_16_c51f8/1 -> Product_ec6fc/2
  Subtract_5712a/1 -> Add_8dc90/1
  Product_ec6fc/1 -> Add_8dc90/2
  Add_8dc90/1 -> Blockout_d_iq_load_16_0762f/1

== system IEEE30_case/AC_1/d_iq_load_17_block ==
  note: d_iq_load_17 in IEEE30_case
      | $78.0853999068988\,\mathrm{vq}_{\mathrm{bus},17}-584.986218254651\,\mathrm{iq}_{\mathrm{load},17}-376.991118430775\,\mathrm{id}_{\mathrm{load},17}$
      | Automatically generated on 2025-11-01 18:40:37 .
  State_id_load_17_33982 : Inport
  State_iq_load_17_00d7f : Inport  Port=2
  State_vq_bus_17_aeaf0 : Inport  Port=3
  Add_f7430 : Sum
  Constant_-376.991118430775_351de : Constant  Value=-376.991118430775
  Constant_584.986218254651_41463 : Constant  Value=584.986218254651
  Constant_78.0853999068988_2afd1 : Constant  Value=78.0853999068988
  Product_19578 : Product
  Product_29a69 : Product
  Product_dc837 : Product
  Subtract_de1c4 : Sum  Inputs=+-
  Blockout_d_iq_load_17_3c8b9 : Outport
  wires:
  Constant_-376.991118430775_351de/1 -> Product_29a69/1
  Constant_584.986218254651_41463/1 -> Product_dc837/1
  Product_dc837/1 -> Subtract_de1c4/2
  State_id_load_17_33982/1 -> Product_29a69/2
  State_iq_load_17_00d7f/1 -> Product_dc837/2
  Product_29a69/1 -> Subtract_de1c4/1
  Constant_78.0853999068988_2afd1/1 -> Product_19578/1
  State_vq_bus_17_aeaf0/1 -> Product_19578/2
  Subtract_de1c4/1 -> Add_f7430/1
  Product_19578/1 -> Add_f7430/2
  Add_f7430/1 -> Blockout_d_iq_load_17_3c8b9/1

== system IEEE30_case/AC_1/d_iq_load_18_block ==
  note: d_iq_load_18 in IEEE30_case
      | $49.3520450041255\,\mathrm{vq}_{\mathrm{bus},18}-1340.41286553164\,\mathrm{iq}_{\mathrm{load},18}-376.991118430775\,\mathrm{id}_{\mathrm{load},18}$
      | Automatically generated on 2025-11-01 18:40:39 .
  State_id_load_18_cc435 : Inport
  State_iq_load_18_d8478 : Inport  Port=2
  State_vq_bus_18_1cdbe : Inport  Port=3
  Add_6fb2f : Sum
  Constant_-376.991118430775_f2fe2 : Constant  Value=-376.991118430775
  Constant_1340.41286553164_f73e8 : Constant  Value=1340.41286553164
  Constant_49.3520450041255_95a9c : Constant  Value=49.3520450041255
  Product_979f9 : Product
  Product_a76e6 : Product
  Product_ccd50 : Product
  Subtract_1e928 : Sum  Inputs=+-
  Blockout_d_iq_load_18_ea1d4 : Outport
  wires:
  State_id_load_18_cc435/1 -> Product_979f9/2
  Constant_-376.991118430775_f2fe2/1 -> Product_979f9/1
  Constant_1340.41286553164_f73e8/1 -> Product_ccd50/1
  Product_ccd50/1 -> Subtract_1e928/2
  State_iq_load_18_d8478/1 -> Product_ccd50/2
  Product_979f9/1 -> Subtract_1e928/1
  Constant_49.3520450041255_95a9c/1 -> Product_a76e6/1
  State_vq_bus_18_1cdbe/1 -> Product_a76e6/2
  Subtract_1e928/1 -> Add_6fb2f/1
  Product_a76e6/1 -> Add_6fb2f/2
  Add_6fb2f/1 -> Blockout_d_iq_load_18_ea1d4/1

== system IEEE30_case/AC_1/d_iq_load_19_block ==
  note: d_iq_load_19 in IEEE30_case
      | $121.151749063551\,\mathrm{vq}_{\mathrm{bus},19}-1053.35753679187\,\mathrm{iq}_{\mathrm{load},19}-376.991118430775\,\mathrm{id}_{\mathrm{load},19}$
      | Automatically generated on 2025-11-01 18:40:41 .
  State_id_load_19_a4f80 : Inport
  State_iq_load_19_a3943 : Inport  Port=2
  State_vq_bus_19_94ea2 : Inport  Port=3
  Add_410b9 : Sum
  Constant_-376.991118430775_f8b2f : Constant  Value=-376.991118430775
  Constant_1053.35753679187_737a4 : Constant  Value=1053.35753679187
  Constant_121.151749063551_5e61c : Constant  Value=121.151749063551
  Product_09819 : Product
  Product_8d40b : Product
  Product_8ed21 : Product
  Subtract_dd1ff : Sum  Inputs=+-
  Blockout_d_iq_load_19_8f082 : Outport
  wires:
  Constant_-376.991118430775_f8b2f/1 -> Product_8d40b/1
  State_id_load_19_a4f80/1 -> Product_8d40b/2
  Constant_1053.35753679187_737a4/1 -> Product_8ed21/1
  Product_8ed21/1 -> Subtract_dd1ff/2
  State_iq_load_19_a3943/1 -> Product_8ed21/2
  Product_8d40b/1 -> Subtract_dd1ff/1
  Constant_121.151749063551_5e61c/1 -> Product_09819/1
  State_vq_bus_19_94ea2/1 -> Product_09819/2
  Subtract_dd1ff/1 -> Add_410b9/1
  Product_09819/1 -> Add_410b9/2
  Add_410b9/1 -> Blockout_d_iq_load_19_8f082/1

== system IEEE30_case/AC_1/d_iq_load_20_block ==
  note: d_iq_load_20 in IEEE30_case
      | $30.5607236833912\,\mathrm{vq}_{\mathrm{bus},20}-1184.82922935387\,\mathrm{iq}_{\mathrm{load},20}-376.991118430775\,\mathrm{id}_{\mathrm{load},20}$
      | Automatically generated on 2025-11-01 18:40:43 .
  State_id_load_20_a93db : Inport
  State_iq_load_20_f0103 : Inport  Port=2
  State_vq_bus_20_5757f : Inport  Port=3
  Add_5fbfa : Sum
  Constant_-376.991118430775_98607 : Constant  Value=-376.991118430775
  Constant_1184.82922935387_99242 : Constant  Value=1184.82922935387
  Constant_30.5607236833912_655b2 : Constant  Value=30.5607236833912
  Product_1073e : Product
  Product_bcc77 : Product
  Product_fabfb : Product
  Subtract_cfad3 : Sum  Inputs=+-
  Blockout_d_iq_load_20_f0a03 : Outport
  wires:
  Constant_-376.991118430775_98607/1 -> Product_fabfb/1
  Constant_30.5607236833912_655b2/1 -> Product_bcc77/1
  State_id_load_20_a93db/1 -> Product_fabfb/2
  Constant_1184.82922935387_99242/1 -> Product_1073e/1
  Product_1073e/1 -> Subtract_cfad3/2
  Product_fabfb/1 -> Subtract_cfad3/1
  State_iq_load_20_f0103/1 -> Product_1073e/2
  State_vq_bus_20_5757f/1 -> Product_bcc77/2
  Subtract_cfad3/1 -> Add_5fbfa/1
  Product_bcc77/1 -> Add_5fbfa/2
  Add_5fbfa/1 -> Blockout_d_iq_load_20_f0a03/1

== system IEEE30_case/AC_1/d_iq_load_21_block ==
  note: d_iq_load_21 in IEEE30_case
      | $147.248668081812\,\mathrm{vq}_{\mathrm{bus},21}-589.048622548086\,\mathrm{iq}_{\mathrm{load},21}-376.991118430775\,\mathrm{id}_{\mathrm{load},21}$
      | Automatically generated on 2025-11-01 18:40:45 .
  State_id_load_21_1a39e : Inport
  State_iq_load_21_200f9 : Inport  Port=2
  State_vq_bus_21_cc767 : Inport  Port=3
  Add_47351 : Sum
  Constant_-376.991118430775_620ea : Constant  Value=-376.991118430775
  Constant_147.248668081812_ce267 : Constant  Value=147.248668081812
  Constant_589.048622548086_e8725 : Constant  Value=589.048622548086
  Product_409a9 : Product
  Product_8acc8 : Product
  Product_f535b : Product
  Subtract_8b118 : Sum  Inputs=+-
  Blockout_d_iq_load_21_5945b : Outport
  wires:
  Constant_-376.991118430775_620ea/1 -> Product_8acc8/1
  Constant_589.048622548086_e8725/1 -> Product_409a9/1
  Product_409a9/1 -> Subtract_8b118/2
  State_id_load_21_1a39e/1 -> Product_8acc8/2
  State_iq_load_21_200f9/1 -> Product_409a9/2
  Product_8acc8/1 -> Subtract_8b118/1
  Constant_147.248668081812_ce267/1 -> Product_f535b/1
  State_vq_bus_21_cc767/1 -> Product_f535b/2
  Subtract_8b118/1 -> Add_47351/1
  Product_f535b/1 -> Add_47351/2
  Add_47351/1 -> Blockout_d_iq_load_21_5945b/1

== system IEEE30_case/AC_1/d_iq_load_23_block ==
  note: d_iq_load_23 in IEEE30_case
      | $30.159289474462\,\mathrm{vq}_{\mathrm{bus},23}-753.98223686155\,\mathrm{iq}_{\mathrm{load},23}-376.991118430775\,\mathrm{id}_{\mathrm{load},23}$
      | Automatically generated on 2025-11-01 18:40:47 .
  State_id_load_23_359e1 : Inport
  State_iq_load_23_3c73d : Inport  Port=2
  State_vq_bus_23_fbc77 : Inport  Port=3
  Add_6b46f : Sum
  Constant_-376.991118430775_dc465 : Constant  Value=-376.991118430775
  Constant_30.159289474462_b946c : Constant  Value=30.159289474462
  Constant_753.98223686155_8a743 : Constant  Value=753.98223686155
  Product_11717 : Product
  Product_6b2be : Product
  Product_fb170 : Product
  Subtract_657dd : Sum  Inputs=+-
  Blockout_d_iq_load_23_36f94 : Outport
  wires:
  State_id_load_23_359e1/1 -> Product_11717/2
  Constant_-376.991118430775_dc465/1 -> Product_11717/1
  Constant_753.98223686155_8a743/1 -> Product_6b2be/1
  Product_6b2be/1 -> Subtract_657dd/2
  State_iq_load_23_3c73d/1 -> Product_6b2be/2
  Product_11717/1 -> Subtract_657dd/1
  Constant_30.159289474462_b946c/1 -> Product_fb170/1
  State_vq_bus_23_fbc77/1 -> Product_fb170/2
  Subtract_657dd/1 -> Add_6b46f/1
  Product_fb170/1 -> Add_6b46f/2
  Add_6b46f/1 -> Blockout_d_iq_load_23_36f94/1

== system IEEE30_case/AC_1/d_iq_load_24_block ==
  note: d_iq_load_24 in IEEE30_case
      | $69.4256561190419\,\mathrm{vq}_{\mathrm{bus},24}-489.525780648917\,\mathrm{iq}_{\mathrm{load},24}-376.991118430775\,\mathrm{id}_{\mathrm{load},24}$
      | Automatically generated on 2025-11-01 18:40:49 .
  State_id_load_24_9d769 : Inport
  State_iq_load_24_562ce : Inport  Port=2
  State_vq_bus_24_612f6 : Inport  Port=3
  Add_13a83 : Sum
  Constant_-376.991118430775_b699c : Constant  Value=-376.991118430775
  Constant_489.525780648917_d5465 : Constant  Value=489.525780648917
  Constant_69.4256561190419_dd8cc : Constant  Value=69.4256561190419
  Product_2ee25 : Product
  Product_3a6de : Product
  Product_40715 : Product
  Subtract_c28d0 : Sum  Inputs=+-
  Blockout_d_iq_load_24_ad216 : Outport
  wires:
  Constant_-376.991118430775_b699c/1 -> Product_3a6de/1
  State_id_load_24_9d769/1 -> Product_3a6de/2
  Constant_489.525780648917_d5465/1 -> Product_2ee25/1
  Product_2ee25/1 -> Subtract_c28d0/2
  State_iq_load_24_562ce/1 -> Product_2ee25/2
  Product_3a6de/1 -> Subtract_c28d0/1
  Constant_69.4256561190419_dd8cc/1 -> Product_40715/1
  State_vq_bus_24_612f6/1 -> Product_40715/2
  Subtract_c28d0/1 -> Add_13a83/1
  Product_40715/1 -> Add_13a83/2
  Add_13a83/1 -> Blockout_d_iq_load_24_ad216/1

== system IEEE30_case/AC_1/d_iq_load_26_block ==
  note: d_iq_load_26 in IEEE30_case
      | $30.4177344988829\,\mathrm{vq}_{\mathrm{bus},26}-573.682136742484\,\mathrm{iq}_{\mathrm{load},26}-376.991118430775\,\mathrm{id}_{\mathrm{load},26}$
      | Automatically generated on 2025-11-01 18:40:51 .
  State_id_load_26_7e9e7 : Inport
  State_iq_load_26_73904 : Inport  Port=2
  State_vq_bus_26_a53b6 : Inport  Port=3
  Add_d2495 : Sum
  Constant_-376.991118430775_df83b : Constant  Value=-376.991118430775
  Constant_30.4177344988829_697d1 : Constant  Value=30.4177344988829
  Constant_573.682136742484_71e79 : Constant  Value=573.682136742484
  Product_11220 : Product
  Product_3e98e : Product
  Product_b2e98 : Product
  Subtract_c090a : Sum  Inputs=+-
  Blockout_d_iq_load_26_2c5ef : Outport
  wires:
  Constant_-376.991118430775_df83b/1 -> Product_3e98e/1
  Constant_30.4177344988829_697d1/1 -> Product_b2e98/1
  State_id_load_26_7e9e7/1 -> Product_3e98e/2
  Constant_573.682136742484_71e79/1 -> Product_11220/1
  Product_11220/1 -> Subtract_c090a/2
  State_iq_load_26_73904/1 -> Product_11220/2
  Product_3e98e/1 -> Subtract_c090a/1
  State_vq_bus_26_a53b6/1 -> Product_b2e98/2
  Subtract_c090a/1 -> Add_d2495/1
  Product_b2e98/1 -> Add_d2495/2
  Add_d2495/1 -> Blockout_d_iq_load_26_2c5ef/1

== system IEEE30_case/AC_1/d_iq_load_29_block ==
  note: d_iq_load_29 in IEEE30_case
      | $28.6786928048477\,\mathrm{vq}_{\mathrm{bus},29}-1005.30964914873\,\mathrm{iq}_{\mathrm{load},29}-376.991118430775\,\mathrm{id}_{\mathrm{load},29}$
      | Automatically generated on 2025-11-01 18:40:53 .
  State_id_load_29_0ee5a : Inport
  State_iq_load_29_c7734 : Inport  Port=2
  State_vq_bus_29_603a8 : Inport  Port=3
  Add_76adb : Sum
  Constant_-376.991118430775_19b6d : Constant  Value=-376.991118430775
  Constant_1005.30964914873_83105 : Constant  Value=1005.30964914873
  Constant_28.6786928048477_20e1d : Constant  Value=28.6786928048477
  Product_5299e : Product
  Product_b156c : Product
  Product_f6353 : Product
  Subtract_cf4d7 : Sum  Inputs=+-
  Blockout_d_iq_load_29_f93a9 : Outport
  wires:
  Constant_-376.991118430775_19b6d/1 -> Product_f6353/1
  State_id_load_29_0ee5a/1 -> Product_f6353/2
  Constant_1005.30964914873_83105/1 -> Product_5299e/1
  Product_5299e/1 -> Subtract_cf4d7/2
  State_iq_load_29_c7734/1 -> Product_5299e/2
  Product_f6353/1 -> Subtract_cf4d7/1
  Constant_28.6786928048477_20e1d/1 -> Product_b156c/1
  State_vq_bus_29_603a8/1 -> Product_b156c/2
  Subtract_cf4d7/1 -> Add_76adb/1
  Product_b156c/1 -> Add_76adb/2
  Add_76adb/1 -> Blockout_d_iq_load_29_f93a9/1

== system IEEE30_case/AC_1/d_iq_load_2_block ==
  note: d_iq_load_2 in IEEE30_case
      | $187.658460826431\,\mathrm{vq}_{\mathrm{bus},2}-644.150178736049\,\mathrm{iq}_{\mathrm{load},2}-376.991118430775\,\mathrm{id}_{\mathrm{load},2}$
      | Automatically generated on 2025-11-01 18:40:15 .
  State_id_load_2_4fe58 : Inport
  State_iq_load_2_ec1f4 : Inport  Port=2
  State_vq_bus_2_2efc8 : Inport  Port=3
  Add_30724 : Sum
  Constant_-376.991118430775_e334a : Constant  Value=-376.991118430775
  Constant_187.658460826431_3f77f : Constant  Value=187.658460826431
  Constant_644.150178736049_896e9 : Constant  Value=644.150178736049
  Product_cd4ff : Product
  Product_e1693 : Product
  Product_fd6a0 : Product
  Subtract_f416b : Sum  Inputs=+-
  Blockout_d_iq_load_2_69c38 : Outport
  wires:
  Constant_-376.991118430775_e334a/1 -> Product_fd6a0/1
  State_id_load_2_4fe58/1 -> Product_fd6a0/2
  Constant_644.150178736049_896e9/1 -> Product_e1693/1
  Product_e1693/1 -> Subtract_f416b/2
  State_iq_load_2_ec1f4/1 -> Product_e1693/2
  Product_fd6a0/1 -> Subtract_f416b/1
  Constant_187.658460826431_3f77f/1 -> Product_cd4ff/1
  State_vq_bus_2_2efc8/1 -> Product_cd4ff/2
  Subtract_f416b/1 -> Add_30724/1
  Product_cd4ff/1 -> Add_30724/2
  Add_30724/1 -> Blockout_d_iq_load_2_69c38/1

== system IEEE30_case/AC_1/d_iq_load_30_block ==
  note: d_iq_load_30 in IEEE30_case
      | $245.627822821845\,\mathrm{vq}_{\mathrm{bus},30}-2103.21360808748\,\mathrm{iq}_{\mathrm{load},30}-376.991118430775\,\mathrm{id}_{\mathrm{load},30}$
      | Automatically generated on 2025-11-01 18:40:55 .
  State_id_load_30_df562 : Inport
  State_iq_load_30_a149a : Inport  Port=2
  State_vq_bus_30_d32ca : Inport  Port=3
  Add_c535f : Sum
  Constant_-376.991118430775_570b4 : Constant  Value=-376.991118430775
  Constant_2103.21360808748_26ae3 : Constant  Value=2103.21360808748
  Constant_245.627822821845_ccf42 : Constant  Value=245.627822821845
  Product_685a2 : Product
  Product_a2648 : Product
  Product_c733e : Product
  Subtract_4b140 : Sum  Inputs=+-
  Blockout_d_iq_load_30_29807 : Outport
  wires:
  Constant_-376.991118430775_570b4/1 -> Product_c733e/1
  Constant_245.627822821845_ccf42/1 -> Product_685a2/1
  State_id_load_30_df562/1 -> Product_c733e/2
  Constant_2103.21360808748_26ae3/1 -> Product_a2648/1
  Product_a2648/1 -> Subtract_4b140/2
  State_iq_load_30_a149a/1 -> Product_a2648/2
  Product_c733e/1 -> Subtract_4b140/1
  State_vq_bus_30_d32ca/1 -> Product_685a2/2
  Subtract_4b140/1 -> Add_c535f/1
  Product_685a2/1 -> Add_c535f/2
  Add_c535f/1 -> Blockout_d_iq_load_30_29807/1

== system IEEE30_case/AC_1/d_iq_load_3_block ==
  note: d_iq_load_3 in IEEE30_case
      | $23.4020092990225\,\mathrm{vq}_{\mathrm{bus},3}-753.98223686155\,\mathrm{iq}_{\mathrm{load},3}-376.991118430775\,\mathrm{id}_{\mathrm{load},3}$
      | Automatically generated on 2025-11-01 18:40:18 .
  State_id_load_3_67436 : Inport
  State_iq_load_3_5e9df : Inport  Port=2
  State_vq_bus_3_cb59e : Inport  Port=3
  Add_384b8 : Sum
  Constant_-376.991118430775_2c1a1 : Constant  Value=-376.991118430775
  Constant_23.4020092990225_8862a : Constant  Value=23.4020092990225
  Constant_753.98223686155_33442 : Constant  Value=753.98223686155
  Product_224db : Product
  Product_36204 : Product
  Product_9daa5 : Product
  Subtract_42e46 : Sum  Inputs=+-
  Blockout_d_iq_load_3_3c3bc : Outport
  wires:
  Constant_-376.991118430775_2c1a1/1 -> Product_224db/1
  Constant_23.4020092990225_8862a/1 -> Product_36204/1
  State_id_load_3_67436/1 -> Product_224db/2
  Constant_753.98223686155_33442/1 -> Product_9daa5/1
  Product_9daa5/1 -> Subtract_42e46/2
  State_iq_load_3_5e9df/1 -> Product_9daa5/2
  Product_224db/1 -> Subtract_42e46/1
  State_vq_bus_3_cb59e/1 -> Product_36204/2
  Subtract_42e46/1 -> Add_384b8/1
  Product_36204/1 -> Add_384b8/2
  Add_384b8/1 -> Blockout_d_iq_load_3_3c3bc/1
